simulink model "sf_elevator_old"  (Simulink 7.6)
settings: Solver=FixedStepDiscrete  StartTime=0.0  StopTime=inf  FixedStep=0.01  RelTol=1e-3
InitFcn:
  | allCarIds = [1 2];
StartFcn:
  | sf_elevator_gui('init', 'sf_elevator_old', allCarIds);
StopFcn:
  | sf_elevator_gui('close');
CloseFcn:
  | sf_elevator_gui('close');
  | clear allCarIds;
settings Model: Creator=The MathWorks Inc.  CovMetricSettings=dcmtr  ExtModeAutoUpdateStatusClock=off
settings DataIOCC: SaveFormat=StructureWithTime  SignalLoggingName=sigsOut
settings OptimizationCC: InlineInvariantSignals=on  InitFltsAndDblsToZero=on  EfficientMapNaN2IntZero=off  OptimizeModelRefInitCode=on  LifeSpan=Inf
settings DebuggingCC: SaveWithParameterizedLinksMsg=none  SolverPrmCheckMsg=none  MultiTaskDSMMsg=warning  MultiTaskCondExecSysMsg=none  MultiTaskRateTransMsg=warning  StrictBusMsg=None
settings HardwareCC: TargetUnknown=on
settings SFSimCC: SFSimEnableDebug=off  SFSimOverflowDetection=off  SFSimEcho=off  SimIntegrity=off  SimParseCustomCode=off
settings RTWCC: SystemTargetFile=ert.tlc  TemplateMakefile=ert_default_tmf  Description=Real-Time Workshop Embedded Coder  ProcessScript=ert_make_rtw_hook  IncludeERTFirstTime=on
settings CodeAppCC: IgnoreCustomStorageClasses=off
settings ERTTargetCC: MultiwordLength=2048  GenerateSampleERTMain=on  ERTCustomFileTemplate=example_file_process.tlc  ConvertIfToSwitch=off

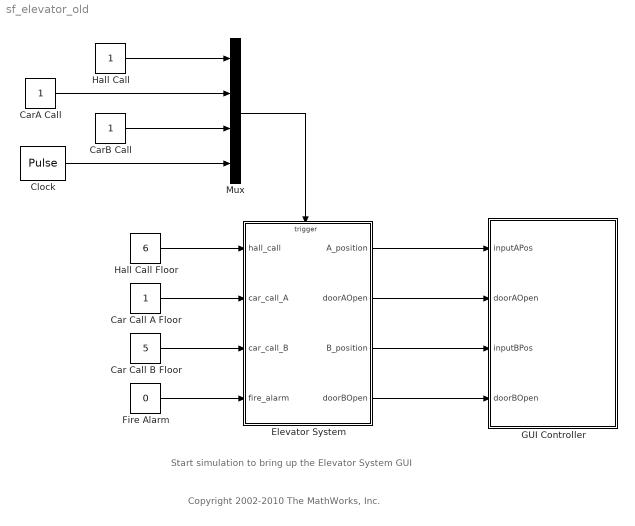
== system sf_elevator_old ==
  note: Start simulation to bring up the Elevator System GUI
  note: Copyright 2002-2010 The MathWorks, Inc.
  Car Call A Floor : Constant  OutDataTypeStr=uint8
  Car Call B Floor : Constant  Value=5  OutDataTypeStr=uint8
  CarA Call : Constant  OutDataTypeStr=double
  CarB Call : Constant  OutDataTypeStr=double
  Clock : DiscretePulseGenerator  PulseType=Time based  PulseWidth=50
  Elevator System : Stateflow chart  TreatAsAtomicUnit=on
  Fire Alarm : Constant  Value=0  OutDataTypeStr=uint8
  GUI Controller : Stateflow chart  TreatAsAtomicUnit=on
  Hall Call : Constant  OutDataTypeStr=double
  Hall Call Floor : Constant  Value=6  OutDataTypeStr=uint8
  Mux : Mux
  wires:
  Hall Call Floor/1 -> Elevator System/1(hall_call)
  Car Call A Floor/1 -> Elevator System/2(car_call_A)
  Car Call B Floor/1 -> Elevator System/3(car_call_B)
  Fire Alarm/1 -> Elevator System/4(fire_alarm)
  Hall Call/1 -> Mux/1
  CarA Call/1 -> Mux/2
  CarB Call/1 -> Mux/3
  Clock/1 -> Mux/4
  Mux/1 -> Elevator System/Trigger
  Elevator System/1(A_position) -> GUI Controller/1(inputAPos)
  Elevator System/2(doorAOpen) -> GUI Controller/2(doorAOpen)
  Elevator System/3(B_position) -> GUI Controller/3(inputBPos)
  Elevator System/4(doorBOpen) -> GUI Controller/4(doorBOpen)

== stateflow chart Elevator System ==
  state Elevator_Manager [parallel]
    du: A_position = Elevator_A.get_position();
    B_position = Elevator_B.get_position();
    settings: executionOrder=1
    state process_hall_call() [function]
      (default) -> (junction 161)
      (junction 161) -> (junction 162) : {
          | /* 'INIT':Initialization */
          | request_floor = hall_call_queue[0];
          | }
      (junction 162) -> (junction 163) : {
          | /* Fire alarm is on */
          | fire_alarm_on = (fire_alarm);
          | }
      (junction 163) -> (junction 164) : {
          | /* There is outstanding request */
          | request_outstanding = (request_floor > 0);
          | }
      (junction 164) -> (junction 165) : {
          | /* Elevator A is idle */
          | elevator_A_idle = (Elevator_A.get_status() == IDLE);
          | }
      (junction 165) -> (junction 166) : {
          | /* Elevator B is idle */
          | elevator_B_idle = (Elevator_B.get_status() == IDLE);
          | }
      (junction 166) -> (junction 167) : {
          | /* Elevator A is closer to request */
          | elevator_A_closer = (fabs(Elevator_A.get_position() - request_floor) <= fabs(Elevator_B.get_position() - request_floor));
          | }
      (junction 167) -> (junction 168) [order 1] : [fire_alarm_on]
      (junction 168) -> (junction 169) : {
          | /* 'EMR':Emergency */
          | Elevator_A.register(floor(Elevator_A.get_position()+Elevator_A.get_direction()/2));
          | Elevator_B.register(floor(Elevator_B.get_position()+Elevator_B.get_direction()/2));
          | }
      (junction 167) -> (junction 170) [order 2]
      (junction 170) -> (junction 171) [order 1] : [!request_outstanding]
      (junction 171) -> (junction 172) : {
          | /* 'NONE':Both elevators are busy or no request present */
          |
          | }
      (junction 170) -> (junction 173) [order 2]
      (junction 173) -> (junction 174) [order 1] : [!elevator_A_idle && !elevator_B_idle]
      (junction 174) -> (junction 175) : {
          | /* 'NONE':Both elevators are busy or no request present */
          |
          | }
      (junction 173) -> (junction 176) [order 2]
      (junction 176) -> (junction 177) [order 1] : [elevator_A_idle && !elevator_B_idle]
      (junction 177) -> (junction 178) : {
          | /* 'A':Elevator A should respond to request */
          | Elevator_A.enqueue(request_floor);
          | dequeue(request_floor);
          | }
      (junction 176) -> (junction 179) [order 2]
      (junction 179) -> (junction 180) [order 1] : [!elevator_A_idle && elevator_B_idle]
      (junction 180) -> (junction 181) : {
          | /* 'B':Elevator B should respond to request */
          | Elevator_B.enqueue(request_floor);
          | dequeue(request_floor);
          | }
      (junction 179) -> (junction 182) [order 2]
      (junction 182) -> (junction 183) [order 1] : [elevator_A_idle && elevator_B_idle && elevator_A_closer]
      (junction 183) -> (junction 184) : {
          | /* 'A':Elevator A should respond to request */
          | Elevator_A.enqueue(request_floor);
          | dequeue(request_floor);
          | }
      (junction 182) -> (junction 185) [order 2]
      (junction 185) -> (junction 186) [order 1] : [elevator_A_idle && elevator_B_idle && !elevator_A_closer]
      (junction 186) -> (junction 187) : {
          | /* 'B':Elevator B should respond to request */
          | Elevator_B.enqueue(request_floor);
          | dequeue(request_floor);
          | }
      (junction 185) -> (junction 188) [order 2]
    state deregister(hall_call_floor) [function]
      (default) -> (junction 106) : {dequeue(hall_call_floor);
          | hall_call_status[hall_call_floor] = 0;}
    state enqueue(hall_call_floor) [function]
      (junction 51) -> (junction 50) [order 1] : [hall_call_status[hall_call_floor] != 0]
      (default) -> (junction 51)
      (junction 66) -> (junction 61) [order 1] : [i >= NUM_FLOOR]
      (junction 66) -> (junction 62) [order 2] : {hall_call_queue[i] = hall_call_floor;}
      (junction 68) -> (junction 66) [order 3]
      (junction 68) -> (junction 68) [order 2] : [hall_call_queue[i] > 0 && i<NUM_FLOOR]{i++;}
      (junction 68) -> (junction 67) [order 1] : [hall_call_queue[i] == hall_call_floor]
      (junction 51) -> (junction 68) [order 2] : {i = 0;}
    state dequeue(hall_call_floor) [function]
      (junction 46) -> (junction 40) [order 2]
      (junction 46) -> (junction 45) [order 1] : [i >= NUM_FLOOR || hall_call_queue[i] == 0]
      (junction 65) -> (junction 65) [order 1] : [hall_call_queue[i] > 0 && ...
          | i<NUM_FLOOR && ...
          | hall_call_queue[i] != hall_call_floor]{i++;}
      (junction 65) -> (junction 46) [order 2]
      (default) -> (junction 65) : {i=0;}
      (junction 40) -> (junction 64) : {hall_call_queue[i] = hall_call_queue[i+1]; i++;}
      (junction 64) -> (junction 40) [order 1] : [i < NUM_FLOOR]
      (junction 64) -> (junction 108) [order 2]
    state register(hall_call_floor) [function]
      (default) -> (junction 103) : {enqueue(hall_call_floor);
          | hall_call_status[hall_call_floor] = 1;}
    state ans = exists_in_queue(floor) [function]
      (junction 137) -> (junction 135) [order 2] : {ans = i+1;}
      (junction 138) -> (junction 138) [order 1] : [hall_call_queue[i] > 0 && ...
          | i<NUM_FLOOR && ...
          | hall_call_queue[i] != floor]{i++;}
      (junction 138) -> (junction 137) [order 2]
      (junction 137) -> (junction 136) [order 1] : [i >= NUM_FLOOR || hall_call_queue[i] == 0]{ans = 0;}
      (default) -> (junction 138) : {i=0;}
    Elevator_Manager -> (junction 72) [order 1] : CAR_CALL_B{Elevator_B.register(car_call_B);}
    Elevator_Manager -> (junction 73) [order 2] : CAR_CALL_A{Elevator_A.register(car_call_A);}
    Elevator_Manager -> (junction 63) [order 3] : HALL_CALL{register(hall_call);}
    Elevator_Manager -> (junction 54) [order 4] : CLOCK {process_hall_call();}
  state Elevator_A [parallel]
    settings: executionOrder=2
    state stat = get_status() [function]
      (default) -> (junction 43) : {stat = status;}
    state pos = get_position() [function]
      (default) -> (junction 44) : {pos = position;}
    state register(car_call_floor) [function]
      (default) -> (junction 104) : {enqueue(car_call_floor);
          | car_call_status[car_call_floor] = 1;}
    state deregister(car_call_floor) [function]
      (default) -> (junction 105) : {dequeue(car_call_floor);
          | car_call_status[car_call_floor] = 0;}
    state Idle
      en: status = IDLE;
      ex: status = BUSY;
    state dequeue(task_floor) [function]
      (junction 41) -> (junction 69) [order 1] : [i >= NUM_FLOOR || task_queue[i] == 0]
      (junction 42) -> (junction 41) [order 2]
      (junction 42) -> (junction 42) [order 1] : [task_queue[i] > 0 && ...
          | i<NUM_FLOOR && ...
          | task_queue[i] != task_floor]{i++;}
      (default) -> (junction 42) : {i=0;}
      (junction 41) -> (junction 70) [order 2]
      (junction 70) -> (junction 52) : {task_queue[i] = task_queue[i+1]; i++;}
      (junction 52) -> (junction 70) [order 1] : [i < NUM_FLOOR]
      (junction 52) -> (junction 107) [order 2]
    state MoveToTask
      du: move_to(task_queue[0]);
    state PickUpDropOff
      en: Elevator_Manager.deregister(cur_floor);
      deregister(cur_floor);
      direction = MOVE_IDLE;
      doorAOpen = 1;
      du: Elevator_Manager.deregister(cur_floor);
      deregister(cur_floor);
      ex: doorAOpen = 0;
      state Stopped
      Elevator_A.PickUpDropOff.Stopped -> Elevator_A.PickUpDropOff.Stopped [order 2] : [fire_alarm]{status = EMERG;}
          | /* Resets the timeout counter */
    state move_to(destination) [function]
      (junction 87) -> (junction 84) [order 2]
      (junction 86) -> (junction 85) : {
          | /* Move down */
          | position = position - VELOCITY;
          | direction = MOVE_DOWN;
          | }
      (junction 87) -> (junction 86) [order 1] : [!move_up && move_down]
      (junction 90) -> (junction 87) [order 2]
      (junction 89) -> (junction 88) : {
          | /* Move up */
          | position = position + VELOCITY;
          | direction = MOVE_UP;
          | }
      (junction 90) -> (junction 89) [order 1] : [move_up && !move_down]
      (junction 91) -> (junction 90) : {
          | /* Move down */
          | move_down = (position - destination > ERR_TOR);
          | }
      (junction 92) -> (junction 91) : {
          | /* Move up */
          | move_up = (destination - position > ERR_TOR);
          | }
      (default) -> (junction 92)
    state enqueue(task_floor) [function]
      (junction 49) -> (junction 48) [order 1] : [car_call_status[task_floor] != 0]
      (default) -> (junction 49)
      (junction 58) -> (junction 47) [order 2] : {task_queue[i] = task_floor;}
      (junction 58) -> (junction 57) [order 1] : [i >= NUM_FLOOR]
      (junction 59) -> (junction 58) [order 3]
      (junction 59) -> (junction 59) [order 2] : [task_queue[i] > 0 && i<NUM_FLOOR]{i++;}
      (junction 59) -> (junction 60) [order 1] : [task_queue[i] == task_floor]
      (junction 49) -> (junction 59) [order 2] : {i = 0;}
    state ans = should_stop() [function]
      (default) -> (junction 113)
      (junction 113) -> (junction 124) : {
          | /* 'INIT':Initialization */
          | cur_floor = ml_round(position);
          | }
      (junction 124) -> (junction 125) : {
          | /* Arrived destination */
          | at_destination = (fabs(position - task_queue[0]) < ERR_TOR);
          | }
      (junction 125) -> (junction 126) : {
          | /* Arrived a floor */
          | at_a_floor = (fabs(position - cur_floor) < ERR_TOR);
          | }
      (junction 126) -> (junction 127) : {
          | /* There is car call to stop at this floor */
          | request_from_car = (car_call_status[cur_floor]);
          | }
      (junction 127) -> (junction 128) : {
          | /* There is hall call from this floor */
          | request_from_hall = (Elevator_Manager.hall_call_status[cur_floor]);
          | }
      (junction 128) -> (junction 129) : {
          | /* This hall call is still outstanding in queue */
          | this_hall_call_outstanding = (Elevator_Manager.exists_in_queue(cur_floor));
          | }
      (junction 129) -> (junction 93) [order 2]
      (junction 93) -> (junction 100) [order 1] : [!at_a_floor]
      (junction 100) -> (junction 101) : {
          | /* 'C':Should not stop, continue */
          | ans = 0;
          | }
      (junction 129) -> (junction 130) [order 1] : [at_destination]
      (junction 130) -> (junction 131) : {
          | /* 'S':Should stop at this floor */
          | position = cur_floor; /* Adjust position */
          | ans = 1;
          | }
      (junction 140) -> (junction 139) : {
          | /* 'C':Should not stop, continue */
          | ans = 0;
          | }
      (junction 141) -> (junction 140) : /* Default */
      (junction 145) -> (junction 141) [order 2]
      (junction 143) -> (junction 142) : {
          | /* 'S':Should stop at this floor */
          | position = cur_floor; /* Adjust position */
          | ans = 1;
          | }
      (junction 145) -> (junction 143) [order 1] : [request_from_hall && this_hall_call_outstanding]
      (junction 154) -> (junction 145) [order 2]
      (junction 147) -> (junction 146) : {
          | /* 'S':Should stop at this floor */
          | position = cur_floor; /* Adjust position */
          | ans = 1;
          | }
      (junction 154) -> (junction 147) [order 1] : [request_from_car]
      (junction 93) -> (junction 154) [order 2]
    state dir = get_direction() [function]
      (default) -> (junction 81) : {dir = direction;}
    (junction 74) -> Elevator_A.Idle [order 2]
    Elevator_A.Idle -> Elevator_A.MoveToTask : [task_queue[0]]
    Elevator_A.MoveToTask -> Elevator_A.PickUpDropOff : [should_stop()]
    Elevator_A.PickUpDropOff.Stopped -> (junction 74) [order 1] : after(TIME_OUT, CLOCK)
    (default) -> Elevator_A.Idle : {doorAOpen = 0;}
    (junction 74) -> Elevator_A.MoveToTask [order 1] : [task_queue[0]]
  state Elevator_B [parallel]
    settings: executionOrder=3
    state PickUpDropOff
      en: Elevator_Manager.deregister(cur_floor);
      deregister(cur_floor);
      direction = MOVE_IDLE;
      doorBOpen = 1;
      du: Elevator_Manager.deregister(cur_floor);
      deregister(cur_floor);
      ex: doorBOpen = 0;
      state Stopped
      Elevator_B.PickUpDropOff.Stopped -> Elevator_B.PickUpDropOff.Stopped [order 2] : [fire_alarm]{status = EMERG;}
          | /* Resets the timeout counter */
    state Idle
      en: status = IDLE;
      ex: status = BUSY;
    state MoveToTask
      du: move_to(task_queue[0]);
    state move_to(destination) [function]
      (default) -> (junction 102)
      (junction 102) -> (junction 148) : {
          | /* Move up */
          | move_up = (destination - position > ERR_TOR);
          | }
      (junction 148) -> (junction 149) : {
          | /* Move down */
          | move_down = (position - destination > ERR_TOR);
          | }
      (junction 149) -> (junction 150) [order 1] : [move_up && !move_down]
      (junction 150) -> (junction 151) : {
          | /* Move up */
          | position = position + VELOCITY;
          | direction = MOVE_UP;
          | }
      (junction 149) -> (junction 152) [order 2]
      (junction 152) -> (junction 153) [order 1] : [!move_up && move_down]
      (junction 153) -> (junction 155) : {
          | /* Move down */
          | position = position - VELOCITY;
          | direction = MOVE_DOWN;
          | }
      (junction 152) -> (junction 156) [order 2]
    state ans = should_stop [function]
      (junction 82) -> (junction 55) : {
          | /* 'C':Should not stop, continue */
          | ans = 0;
          | }
      (junction 94) -> (junction 82) : /* Default */
      (junction 97) -> (junction 94) [order 2]
      (junction 96) -> (junction 95) : {
          | /* 'S':Should stop at this floor */
          | position = cur_floor; /* Adjust position */
          | ans = 1;
          | }
      (junction 97) -> (junction 96) [order 1] : [request_from_hall && this_hall_call_outstanding]
      (junction 114) -> (junction 97) [order 2]
      (junction 99) -> (junction 98) : {
          | /* 'S':Should stop at this floor */
          | position = cur_floor; /* Adjust position */
          | ans = 1;
          | }
      (junction 114) -> (junction 99) [order 1] : [request_from_car]
      (junction 117) -> (junction 114) [order 2]
      (junction 116) -> (junction 115) : {
          | /* 'C':Should not stop, continue */
          | ans = 0;
          | }
      (junction 117) -> (junction 116) [order 1] : [!at_a_floor]
      (junction 120) -> (junction 117) [order 2]
      (junction 119) -> (junction 118) : {
          | /* 'S':Should stop at this floor */
          | position = cur_floor; /* Adjust position */
          | ans = 1;
          | }
      (junction 120) -> (junction 119) [order 1] : [at_destination]
      (junction 121) -> (junction 120) : {
          | /* This hall call is still outstanding in queue */
          | this_hall_call_outstanding = (Elevator_Manager.exists_in_queue(cur_floor));
          | }
      (junction 122) -> (junction 121) : {
          | /* There is hall call from this floor */
          | request_from_hall = (Elevator_Manager.hall_call_status[cur_floor]);
          | }
      (junction 132) -> (junction 122) : {
          | /* There is car call to stop at this floor */
          | request_from_car = (car_call_status[cur_floor]);
          | }
      (junction 133) -> (junction 132) : {
          | /* Arrived a floor */
          | at_a_floor = (fabs(position - cur_floor) < ERR_TOR);
          | }
      (junction 134) -> (junction 133) : {
          | /* Arrived destination */
          | at_destination = (fabs(position - task_queue[0]) < ERR_TOR);
          | }
      (junction 160) -> (junction 134) : {
          | /* 'INIT':Initialization */
          | cur_floor = ml_round(position);
          | }
      (default) -> (junction 160)
    state dir = get_direction [function]
      (default) -> (junction 109) : {dir = direction;}
    state register(car_call_floor) [function]
      (default) -> (junction 110) : {enqueue(car_call_floor);
          | car_call_status[car_call_floor] = 1;}
    state enqueue(task_floor) [function]
      (junction 159) -> (junction 123) [order 1] : [task_queue[i] == task_floor]
      (junction 159) -> (junction 159) [order 2] : [task_queue[i] > 0 && i<NUM_FLOOR]{i++;}
      (junction 159) -> (junction 158) [order 3]
      (junction 158) -> (junction 157) [order 1] : [i >= NUM_FLOOR]
      (junction 158) -> (junction 56) [order 2] : {task_queue[i] = task_floor;}
      (junction 111) -> (junction 159) [order 2] : {i = 0;}
      (junction 111) -> (junction 112) [order 1] : [car_call_status[task_floor] != 0]
      (default) -> (junction 111)
    state pos = get_position [function]
      (default) -> (junction 71) : {pos = position;}
    state deregister(car_call_floor) [function]
      (default) -> (junction 75) : {dequeue(car_call_floor);
          | car_call_status[car_call_floor] = 0;}
    state stat = get_status [function]
      (default) -> (junction 76) : {stat = status;}
    state dequeue(task_floor) [function]
      (junction 83) -> (junction 53) [order 2]
      (junction 83) -> (junction 80) [order 1] : [i < NUM_FLOOR]
      (junction 80) -> (junction 83) : {task_queue[i] = task_queue[i+1]; i++;}
      (junction 78) -> (junction 80) [order 2]
      (junction 78) -> (junction 79) [order 1] : [i >= NUM_FLOOR || task_queue[i] == 0]
      (junction 77) -> (junction 78) [order 2]
      (junction 77) -> (junction 77) [order 1] : [task_queue[i] > 0 && ...
          | i<NUM_FLOOR && ...
          | task_queue[i] != task_floor]{i++;}
      (default) -> (junction 77) : {i=0;}
    (junction 144) -> Elevator_B.Idle [order 2]
    Elevator_B.MoveToTask -> Elevator_B.PickUpDropOff : [should_stop()]
    Elevator_B.Idle -> Elevator_B.MoveToTask : [task_queue[0]]
    (junction 144) -> Elevator_B.MoveToTask [order 1] : [task_queue[0]]
    Elevator_B.PickUpDropOff.Stopped -> (junction 144) [order 1] : after(TIME_OUT, CLOCK)
    (default) -> Elevator_B.Idle : {doorBOpen = 0;}
  data: request_floor temporary uint8; fire_alarm_on temporary boolean =0; request_outstanding temporary boolean =0; elevator_A_idle temporary boolean =0; elevator_B_idle temporary boolean =0; elevator_A_closer temporary boolean =0; hall_call_queue local uint8 size=10; hall_call_status local uint8 size=10; status local Enum: ElevatorStatus =ElevatorStatus.IDLE; position local double =1; task_queue local uint8 size=10; car_call_status local uint8 size=10; cur_floor local uint8; direction local Enum: ElevatorDirection =ElevatorDirection.MOVE_IDLE; stat function_output uint8; pos function_output double; car_call_floor function_input uint8; hall_call_floor function_input uint8; car_call_floor function_input uint8; i temporary uint8; task_floor function_input uint8; hall_call_floor function_input uint8; i temporary uint8; destination function_input double; move_up temporary boolean =0; move_down temporary boolean =0; i temporary uint8; hall_call_floor function_input uint8; task_floor function_input uint8; i temporary uint8; hall_call_floor function_input uint8; ans function_output boolean; at_destination temporary boolean =0; at_a_floor temporary boolean =0; request_from_car temporary boolean =0; request_from_hall temporary boolean =0; this_hall_call_outstanding temporary boolean =0; dir function_output uint8; ans function_output uint8; floor function_input uint8; i temporary uint8; position local double =1; task_queue local uint8 size=10; car_call_status local uint8 size=10; cur_floor local uint8; direction local Enum: ElevatorDirection =ElevatorDirection.MOVE_IDLE; status local Enum: ElevatorStatus =ElevatorStatus.IDLE; destination function_input double; move_up temporary boolean =0; move_down temporary boolean =0; ans function_output boolean; at_destination temporary boolean =0; at_a_floor temporary boolean =0; request_from_car temporary boolean =0; request_from_hall temporary boolean =0; this_hall_call_outstanding temporary boolean =0; dir function_output uint8; car_call_floor function_input uint8; task_floor function_input uint8; i temporary uint8; pos function_output double; car_call_floor function_input uint8; stat function_output uint8; i temporary uint8; task_floor function_input uint8; inputVal function_input double; out function_output double; inputVal function_input double; out function_output double; VELOCITY constant double =0.005; hall_call input uint8; A_position output double =1; doorAOpen output boolean; B_position output double =1; NUM_FLOOR constant uint8 =9; ERR_TOR constant double =0.001; car_call_A input uint8; car_call_B input uint8; fire_alarm input uint8; TIME_OUT constant uint32 =1000; doorBOpen output boolean
  data fire_alarm_on settings: description=Fire alarm is on
  data request_outstanding settings: description=There is outstanding request
  data elevator_A_idle settings: description=Elevator A is idle
  data elevator_B_idle settings: description=Elevator B is idle
  data elevator_A_closer settings: description=Elevator A is closer to request
  data move_up settings: description=Move up
  data move_down settings: description=Move down
  data at_destination settings: description=Arrived destination
  data at_a_floor settings: description=Arrived a floor
  data request_from_car settings: description=There is car call to stop at this floor
  data request_from_hall settings: description=There is hall call from this floor
  data this_hall_call_outstanding settings: description=This hall call is still outstanding in queue
  data move_up settings: description=Move up
  data move_down settings: description=Move down
  data at_destination settings: description=Arrived destination
  data at_a_floor settings: description=Arrived a floor
  data request_from_car settings: description=There is car call to stop at this floor
  data request_from_hall settings: description=There is hall call from this floor
  data this_hall_call_outstanding settings: description=This hall call is still outstanding in queue
  events: HALL_CALL input EITHER_EDGE_EVENT; CAR_CALL_A input EITHER_EDGE_EVENT; CAR_CALL_B input EITHER_EDGE_EVENT; CLOCK input EITHER_EDGE_EVENT
  function out = ml_round(inputVal):
    | function out = ml_round(inputVal)
    | 
    | out = round(inputVal);
  function out = ml_round(inputVal):
    | function out = ml_round(inputVal)
    | 
    | out = round(inputVal);

== stateflow chart GUI Controller ==
  state CarB_Controller [parallel]
    settings: executionOrder=2
    state floorNumber = get_floor_number(pos) [function]
      (default) -> (junction 491) : {floorNumber = ml.round(pos);}
    state deactivate_car_button(pos) [function]
      (default) -> (junction 492) : {floorNum = get_floor_number(pos);
          | ml.sf_elevator_gui('deactivate',allCarIds[1], floorNum);}
    state deactivate_hall_button(pos) [function]
      (default) -> (junction 493) : {floorNum = get_floor_number(pos);
          | ml.sf_elevator_gui('deactivate','hall', floorNum);}
    state move(pos) [function]
      (default) -> (junction 494) : {ml.sf_elevator_gui('move_car', allCarIds[1], pos);}
    state open_door [function]
      (default) -> (junction 495) : {ml.sf_elevator_gui('open_door', allCarIds[1]);}
    state close_door [function]
      (default) -> (junction 496) : {ml.sf_elevator_gui('close_door', allCarIds[1]);}
    CarB_Controller -> (junction 479)
    (junction 479) -> (junction 480) [order 1] : [hasChanged(inputBPos)]
    (junction 479) -> (junction 481) [order 2]
    (junction 480) -> (junction 482) : {move(inputBPos);}
    (junction 482) -> (junction 481)
    (junction 481) -> (junction 483)
    (junction 483) -> (junction 484) [order 1] : [hasChanged(doorBOpen)]
    (junction 484) -> (junction 485)
    (junction 483) -> (junction 487) [order 2]
    (junction 485) -> (junction 486) [order 1] : [doorBOpen]
    (junction 485) -> (junction 488) [order 2] : {close_door();}
    (junction 486) -> (junction 489) : {open_door();}
    (junction 488) -> (junction 487) : {deactivate_hall_button(inputBPos);
        |  deactivate_car_button(inputBPos);}
    (junction 489) -> (junction 488)
    (junction 487) -> (junction 490)
  state CarA_Controller [parallel]
    settings: executionOrder=1
    state deactivate_car_button(pos) [function]
      (default) -> (junction 476) : {floorNum = get_floor_number(pos);
          | ml.sf_elevator_gui('deactivate',allCarIds[0], floorNum);}
    state floorNumber = get_floor_number(pos) [function]
      (default) -> (junction 477) : {floorNumber = ml.round(pos);}
    state deactivate_hall_button(pos) [function]
      (default) -> (junction 478) : {floorNum = get_floor_number(pos);
          | ml.sf_elevator_gui('deactivate','hall', floorNum);}
    state close_door [function]
      (default) -> (junction 473) : {ml.sf_elevator_gui('close_door', allCarIds[0]);}
    state open_door [function]
      (default) -> (junction 474) : {ml.sf_elevator_gui('open_door', allCarIds[0]);}
    state move(pos) [function]
      (default) -> (junction 475) : {ml.sf_elevator_gui('move_car', allCarIds[0], pos);}
    CarA_Controller -> (junction 461)
    (junction 461) -> (junction 462) [order 1] : [hasChanged(inputAPos)]
    (junction 461) -> (junction 463) [order 2]
    (junction 462) -> (junction 464) : {move(inputAPos);}
    (junction 464) -> (junction 463)
    (junction 463) -> (junction 465)
    (junction 465) -> (junction 466) [order 1] : [hasChanged(doorAOpen)]
    (junction 466) -> (junction 467)
    (junction 465) -> (junction 469) [order 2]
    (junction 467) -> (junction 468) [order 1] : [doorAOpen]
    (junction 467) -> (junction 470) [order 2] : {close_door();}
    (junction 468) -> (junction 471) : {open_door();}
    (junction 470) -> (junction 469) : {deactivate_hall_button(inputAPos);
        |  deactivate_car_button(inputAPos);}
    (junction 471) -> (junction 470)
    (junction 469) -> (junction 472)
  data: pos function_input double; floorNum temporary double; pos function_input double; floorNumber function_output double; pos function_input double; floorNum temporary double; pos function_input double; pos function_input double; floorNumber function_output double; pos function_input double; floorNum temporary double; pos function_input double; floorNum temporary double; pos function_input double; inputAPos input double; doorAOpen input double; inputBPos input double; doorBOpen input double; allCarIds parameter uint8 size=2
